simulink model "Traction_Control"  (R2025b)
settings: Solver=VariableStepAuto  StartTime=0.0  StopTime=10.0  RelTol=1e-3
model workspace (MAT data in the model file):
  fz_values = [0 50 100 150 200 250 300 350 400 450 500 550 ... (43 elements, 1x43)]
  k_opt_lut = [0 0 0 0 0 0 0 0 0 0 0 0 ... (4386 elements, 51x2x43)]
  mu_opt_lut = [0 0 0 0 0 0 0 0 0 0 0 0 ... (4386 elements, 51x2x43)]
libraries: slpidlib x1, simulink x1
(part 2 of 2)

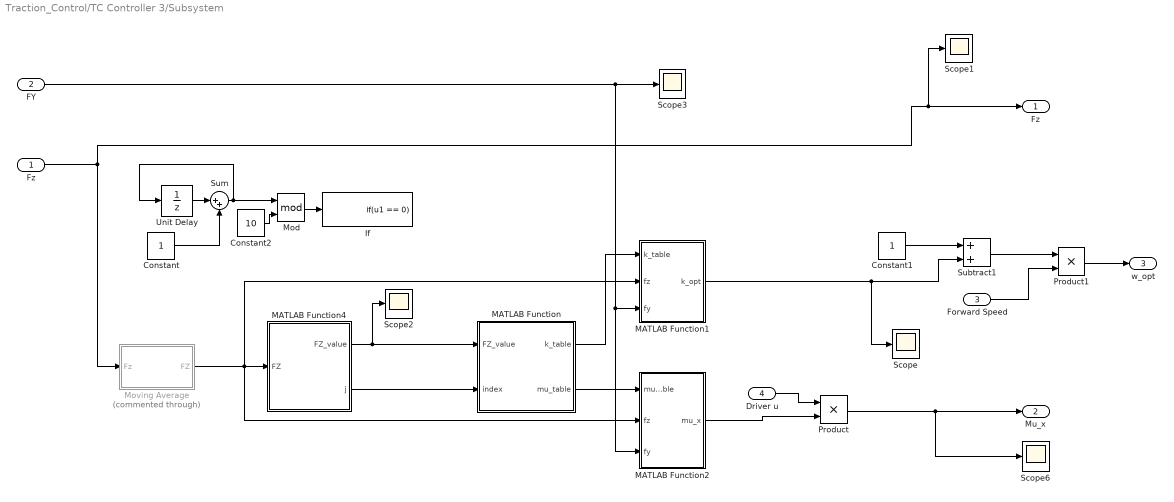
== system Traction_Control/TC Controller 3/Subsystem ==
  "Fz " : Inport
  FY : Inport  Port=2
  Forward Speed : Inport  Port=3
  Driver u : Inport  Port=4
  Constant : Constant
  Constant1 : Constant
  Constant2 : Constant  Value=10
  If : If  IfExpression=u1 == 0  ShowElse=off  ZeroCross=off
  MATLAB Function : MATLAB Function  TreatAsAtomicUnit=on
  MATLAB Function1 : MATLAB Function  TreatAsAtomicUnit=on
  MATLAB Function2 : MATLAB Function  TreatAsAtomicUnit=on
  MATLAB Function4 : MATLAB Function  TreatAsAtomicUnit=on
  Mod : Math  Operator=mod
  Moving Average : Subsystem  Commented=through
  Product : Product
  Product1 : Product
  Scope{,1..3,6} (5 alike) : Scope
      Scope settings: ActiveDisplayYMinimum=0.01999999999999999  ActiveDisplayYMaximum=0.22  DataLoggingVariableName=ScopeData2
      Scope1 settings: ActiveDisplayYMinimum=0.75253153817947194  ActiveDisplayYMaximum=1.0182161563847538  DataLoggingVariableName=ScopeData3
      Scope2 settings: ActiveDisplayYMinimum=-12.499999999999972  ActiveDisplayYMaximum=1112.5  DataLoggingVariableName=ScopeData12
      Scope3 settings: ActiveDisplayYMinimum=-1.4610585575683306  ActiveDisplayYMaximum=1.5143814179529658  DataLoggingVariableName=ScopeData13
      Scope6 settings: ActiveDisplayYMinimum=0.7805564081300761  ActiveDisplayYMaximum=1.6886164894970306  DataLoggingVariableName=ScopeData22
  Subtract1 : Sum
  Sum : Sum  Inputs=|++
  Unit Delay : UnitDelay  SampleTime=-1  HasFrameUpgradeWarning=on
  Fz : Outport
  Mu_x : Outport  Port=2
  w_opt : Outport  Port=3
  wires:
  Product1/1 -> w_opt/1
  Forward Speed/1 -> Product1/2
  "Fz "/1 -> Moving Average/1("Fz "), Scope1/1, Fz/1
  Constant1/1 -> Subtract1/1
  FY/1 -> MATLAB Function2/3(fy), MATLAB Function1/3(fy), Scope3/1
  Subtract1/1 -> Product1/1
  MATLAB Function4/1(FZ_value) -> MATLAB Function/1(FZ_value), Scope2/1
  MATLAB Function4/2(j) -> MATLAB Function/2(index)
  Sum/1 -> Unit Delay/1, Mod/1
  Unit Delay/1 -> Sum/1
  Constant2/1 -> Mod/2
  Constant/1 -> Sum/2
  Mod/1 -> If/1
  MATLAB Function/1(k_table) -> MATLAB Function1/1(k_table)
  MATLAB Function1/1(k_opt) -> Scope/1, Subtract1/2
  MATLAB Function/2(mu_table) -> MATLAB Function2/1(mu_table)
  Moving Average/1(FZ) -> MATLAB Function1/2(fz), MATLAB Function2/2(fz), MATLAB Function4/1(FZ)
  MATLAB Function2/1(mu_x) -> Product/2
  Driver u/1 -> Product/1
  Product/1 -> Mu_x/1, Scope6/1

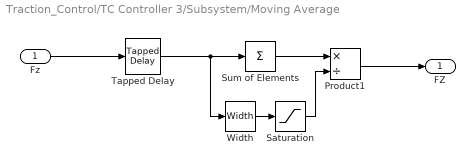
== system Traction_Control/TC Controller 3/Subsystem/Moving Average ==
  "Fz " : Inport
  Product1 : Product  Inputs=*/
  Saturation : Saturate  UpperLimit=inf  LowerLimit=1
  Sum of Elements : Sum  Inputs=+
  Tapped Delay : simulink/Discrete/Tapped Delay  vinit=0.0  samptime=-1  NumDelays=10  DelayOrder=Oldest  includeCurrent=on
  Width : Width
  FZ : Outport
  wires:
  Tapped Delay/1 -> Width/1, Sum of Elements/1
  Sum of Elements/1 -> Product1/1
  Product1/1 -> FZ/1
  "Fz "/1 -> Tapped Delay/1
  Width/1 -> Saturation/1
  Saturation/1 -> Product1/2

== matlab function Traction_Control/TC Controller 3/Subsystem/MATLAB Function ==
  data: FZ_value input; k_table output; index input; mu_table output; k_opt_lut parameter; mu_opt_lut parameter
function [k_table,mu_table] = fcn(FZ_value, index, k_opt_lut, mu_opt_lut)
    k_table = k_opt_lut(:,:,index); 
    mu_table = mu_opt_lut(:,:,index);

== matlab function Traction_Control/TC Controller 3/Subsystem/MATLAB Function1 ==
  data: k_table input; fz input; k_opt output; fy input
function k_opt = fcn(k_table,fz, fy)
    if fz == 0
        k_opt = 0;
    else
        k_opt = interp1(double(k_table(:,1))/10000,double(k_table(:,2))/100,fy,'linear','extrap');
    end

== matlab function Traction_Control/TC Controller 3/Subsystem/MATLAB Function2 ==
  data: mu_table input; fz input; mu_x output; fy input
function mu_x = fcn(mu_table,fz, fy)
    if fz == 0
        mu_x = 0;
    else
        mu_x = interp1(double(mu_table(:,1))/10000,double(mu_table(:,2))/1000,fy,"linear","extrap");
    end

== matlab function Traction_Control/TC Controller 3/MATLAB Function ==
  data: a_y input; F_Y output
function F_Y = fcn(a_y)
m = 250+68; %Mass with driver weight
a = 1.530/2; %Distance cg to front axle with load distribution of 0.5
h = 0.249; %Height of CG
l = 1.530; %Length of wheelbase

F_Y = 0.5*(a/l)*m*a_y;

== matlab function Traction_Control/TC Controller 3/MATLAB Function10 ==
  data: a_x input; F_Z output; a_y input
function F_Z = fcn(a_x, a_y)
m = 250+68; %Mass with driver weight
a = 1.530/2; %Distance cg to front axle with load distribution of 0.5
h = 0.249; %Height of CG
l = 1.530; %Length of wheelbase
tw = 1.2; %Track width
roll_stiffness_r = 0.3482;
F_Z = (1/2)*m*(a+h*a_x)/(l);
%F_Z_out = 1/2*((m*a)/l + (m*h*a_x)/l) + (m*abs(a_y)*h)/tw;
%F_Z_in = 1/2*((m*a)/l + (m*h*a_x)/l) - (m*abs(a_y)*h)/tw;
%F_Z = min(F_Z_out,F_Z_in);

== matlab function Traction_Control/TC Controller 3/Subsystem/MATLAB Function4 ==
  data: FZ input; FZ_value output; j output; fz_values parameter
function [FZ_value,j] = fcn(FZ,fz_values)
  FZ = FZ*1000;
  m = 10000;
  index = 1;
  for i = 1:numel(fz_values)
      delta = abs(FZ - fz_values(i));
      if delta < m
          m = delta;
          index = i;
      else
          m = m;
      end
  end
    FZ_value = fz_values(index);
    j = index;
end
